simulink model "ctrl_ez0"  (R2024b)
settings: Solver=FixedStepDiscrete  StartTime=0.0  StopTime=10.0  RelTol=1e-3  EnableMultiTasking=on
InitFcn:
  | fidelity_pfc_vals;
values from neighbouring files (symbols this model uses):
  cos_th = cos(2*pi*50*t)    [fidelity_pfc_vals.m]
  sin_th = sin(2*pi*50*t)    [fidelity_pfc_vals.m]
  tsw = 1/(fsw*1e3)    (= 1.53846153846e-05)    [fidelity_pfc_vals.m]
undefined symbols (not defined in the file or in its folder): DiscIntNeverNeededParam
libraries: simulink x4, mcbcontrolslib x1, dspswit3 x1, slpidlib x1, simulink_extras x1
settings Model: DataDictionary=dic_pfc3ph.sldd  Creator=Angel  LastModifiedBy=Angel
settings DataIOCC: SaveOutput=off  SaveTime=off
settings OptimizationCC: DefaultParameterBehavior=Inlined  UseDivisionForNetSlopeComputation=on  GainParamInheritBuiltInType=on  UseFloatMulNetSlope=on  DefaultUnderspecifiedDataType=single  InlineInvariantSignals=on  ReuseModelBlockBuffer=off  PassReuseOutputArgsAs=Individual arguments  ZeroExternalMemoryAtStartup=off  ZeroInternalMemoryAtStartup=off  NoFixptDivByZeroProtection=on  EfficientFloat2IntCast=on  LifeSpan=1  BufferReusableBoundary=off  OptimizationLevel=level1  OptimizationPriority=Speed  EfficientTunableParamExpr=on
settings DebuggingCC: MergeDetectMultiDrivingBlocksExec=none  ParameterTunabilityLossMsg=error
settings HardwareCC: ProdBitPerPointer=32  ProdBitPerSizeT=32  ProdBitPerPtrDiffT=32  ProdLargestAtomicInteger=Long  ProdLargestAtomicFloat=Double  ProdWordSize=32  ProdLongLongMode=on  ProdHWDeviceType=ARM Compatible->ARM Cortex-M
settings ModelReferenceCC: ModelReferenceNumInstancesAllowed=Single  PropagateSignalLabelsOutOfModel=off
settings SFSimCC: MATLABDynamicMemAlloc=off
settings RTWCC: Description=Embedded Coder  SystemTargetFile=ert.tlc  EmbeddedCoderDictionary=dic_pfc3ph.sldd  GenCodeOnly=on  TemplateMakefile=ert_default_tmf  Toolchain=CMake  DataTypeReplacement=CDataTypesFixedWidth
settings CodeAppCC: ForceParamTrailComments=on  CommentStyle=Multi-line  IgnoreCustomStorageClasses=off  OperatorAnnotations=on  SimulinkDataObjDesc=on  SFDataObjDesc=on  CustomSymbolStrGlobalVar=rt$N$M  CustomSymbolStrType=$N$M  CustomSymbolStrFcn=$N$M$F  CustomSymbolStrMacro=$N$M  InsertBlockDesc=on
settings ERTTargetCC: IncludeMdlTerminateFcn=off  CombineSignalStateStructs=on  SupportAbsoluteTime=off  SupportComplex=off  SupportNonInlinedSFcns=on  RemoveResetFunc=off  ParenthesesLevel=Standards  RootIOFormat=Structure reference  ERTCustomFileTemplate=example_file_process.tlc  ERTFilePackagingFormat=CompactWithDataFile  MaxIdInt64=INT64_MAX  MinIdInt64=INT64_MIN  MaxIdUint64=UINT64_MAX  MaxIdInt32=INT32_MAX  MinIdInt32=INT32_MIN  MaxIdUint32=UINT32_MAX  MaxIdInt16=INT16_MAX  MinIdInt16=INT16_MIN  MaxIdUint16=UINT16_MAX  MaxIdInt8=INT8_MAX  MinIdInt8=INT8_MIN  MaxIdUint8=UINT8_MAX

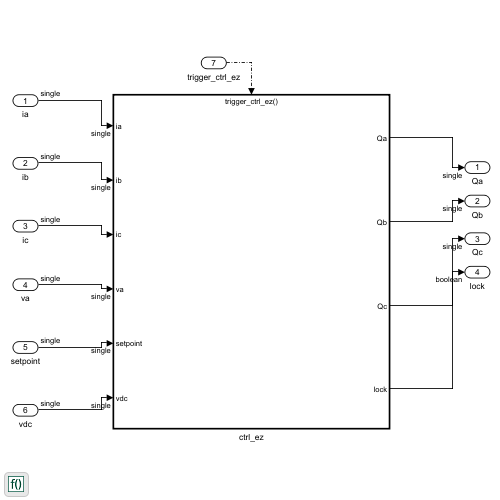
[thumbnail: Simulink's stored preview of the top-level diagram]
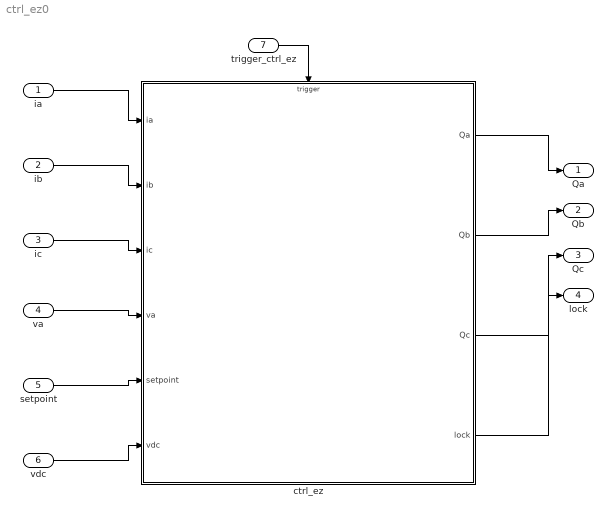
== system ctrl_ez0 ==
  ia : Inport  OutDataTypeStr=single  PortDimensions=1
  ib : Inport  Port=2  OutDataTypeStr=single  PortDimensions=1
  ic : Inport  Port=3  OutDataTypeStr=single  PortDimensions=1
  va : Inport  Port=4  OutDataTypeStr=single  PortDimensions=1
  setpoint : Inport  Port=5  OutDataTypeStr=single  PortDimensions=1
  vdc : Inport  Port=6  OutDataTypeStr=single  PortDimensions=1
  trigger_ctrl_ez : Inport  Port=7  PortDimensions=1  OutputFunctionCall=on
  ctrl_ez : Subsystem
  Qa : Outport  OutDataTypeStr=single  PortDimensions=1
  Qb : Outport  Port=2  OutDataTypeStr=single  PortDimensions=1
  Qc : Outport  Port=3  OutDataTypeStr=single  PortDimensions=1
  lock : Outport  Port=4  OutDataTypeStr=boolean  PortDimensions=1
  wires:
  ia/1 -> ctrl_ez/1(ia)
  ib/1 -> ctrl_ez/2(ib)
  ic/1 -> ctrl_ez/3(ic)
  va/1 -> ctrl_ez/4(va)
  setpoint/1 -> ctrl_ez/5(setpoint)
  vdc/1 -> ctrl_ez/6(vdc)
  ctrl_ez/1(Qa) -> Qa/1
  ctrl_ez/2(Qb) -> Qb/1
  ctrl_ez/3(Qc) -> Qc/1
  ctrl_ez/4(lock) -> lock/1
  trigger_ctrl_ez/1 -> ctrl_ez/Trigger

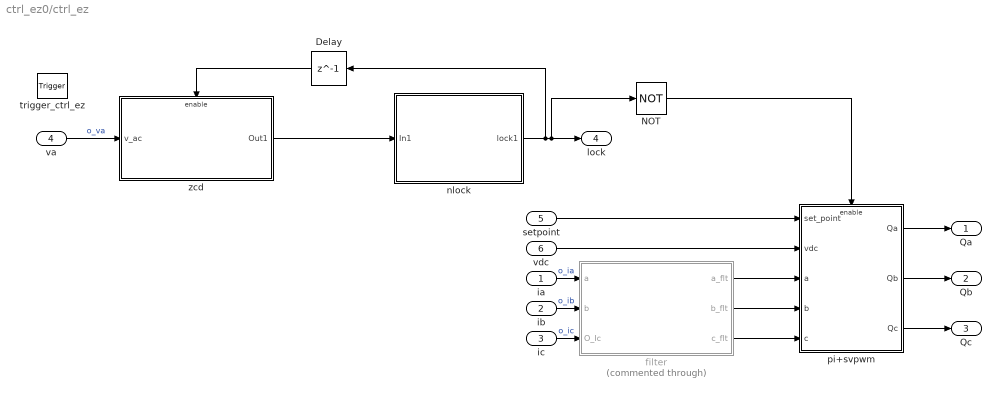
== system ctrl_ez0/ctrl_ez ==
  ia : Inport  OutDataTypeStr=single
  ib : Inport  Port=2  OutDataTypeStr=single
  ic : Inport  Port=3
  va : Inport  Port=4  OutDataTypeStr=single
  setpoint : Inport  Port=5  OutDataTypeStr=single
  vdc : Inport  Port=6  OutDataTypeStr=single
  trigger_ctrl_ez : TriggerPort  TriggerType=function-call  VariantControl=(inherit)  PortDimensions=1
  Delay : Delay  DelayLength=1
  NOT : Logic  Operator=NOT  IconShape=distinctive  AllPortsSameDT=off  OutDataTypeStr=boolean
  filter : Subsystem  Commented=through
  nlock : Subsystem
  pi+svpwm : Subsystem
  zcd : Subsystem  SystemSampleTime=tsw
  Qa : Outport
  Qb : Outport  Port=2
  Qc : Outport  Port=3
  lock : Outport  Port=4
  wires:
  pi+svpwm/3(Qc) -> Qc/1
  pi+svpwm/2(Qb) -> Qb/1
  pi+svpwm/1(Qa) -> Qa/1
  filter/2(b_flt) -> pi+svpwm/4(b)
  vdc/1 -> pi+svpwm/2(vdc)
  setpoint/1 -> pi+svpwm/1(set_point)
  filter/3(c_flt) -> pi+svpwm/5(c)
  nlock/1(lock1) -> Delay/1, NOT/1, lock/1
  zcd/1(Out1) -> nlock/1(In1)
  va/1 -> zcd/1(v_ac)  "o_va"
  filter/1(a_flt) -> pi+svpwm/3(a)
  Delay/1 -> zcd/Enable
  ia/1 -> filter/1(a)  "o_ia"
  ic/1 -> filter/3(O_Ic)  "o_ic"
  NOT/1 -> pi+svpwm/Enable
  ib/1 -> filter/2(b)  "o_ib"

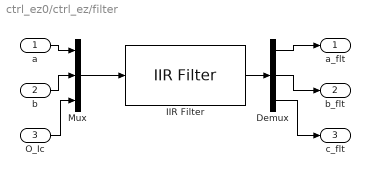
== system ctrl_ez0/ctrl_ez/filter ==
  a : Inport
  b : Inport  Port=2
  O_Ic : Inport  Port=3
  Demux : Demux  Outputs=3
  IIR Filter : mcbcontrolslib/IIR Filter  VariantControl=Low Pass Filter  VariantSelect=Low-pass  FilterConstantInputType=Specify via dialog  Filter_constant=.2  advancedSettings=on  Ts=tsw  cutOff_freq=2586.2678
  Mux : Mux  Inputs=3
  a_flt : Outport
  b_flt : Outport  Port=2
  c_flt : Outport  Port=3
  wires:
  Demux/3 -> c_flt/1
  O_Ic/1 -> Mux/3
  IIR Filter/1 -> Demux/1
  Demux/1 -> a_flt/1
  Mux/1 -> IIR Filter/1
  b/1 -> Mux/2
  Demux/2 -> b_flt/1
  a/1 -> Mux/1

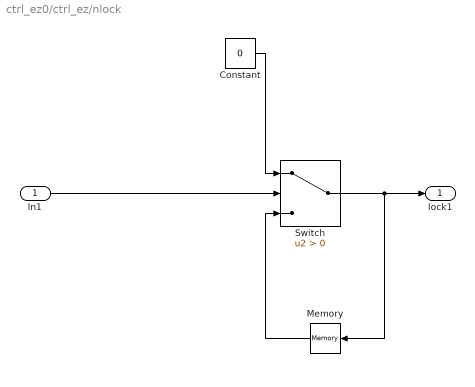
== system ctrl_ez0/ctrl_ez/nlock ==
  In1 : Inport
  Constant : Constant  Value=0  OutDataTypeStr=boolean  SampleTime=-1
  Memory : Memory  InitialCondition=1  InheritSampleTime=on
  Switch : Switch  Criteria=u2 > Threshold  SaturateOnIntegerOverflow=off  InputSameDT=off
  lock1 : Outport
  wires:
  In1/1 -> Switch/2
  Memory/1 -> Switch/3
  Constant/1 -> Switch/1
  Switch/1 -> Memory/1, lock1/1

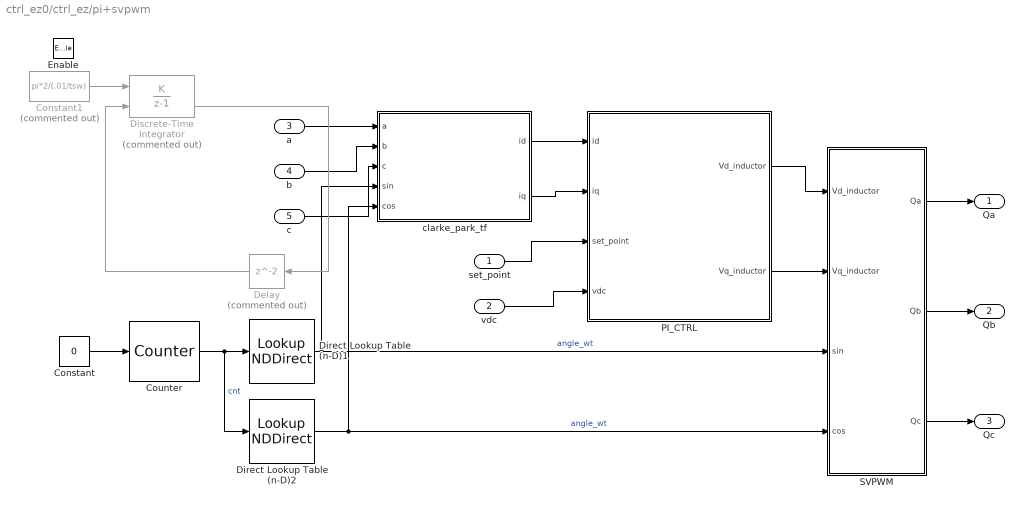
== system ctrl_ez0/ctrl_ez/pi+svpwm ==
  set_point : Inport
  vdc : Inport  Port=2
  a : Inport  Port=3
  b : Inport  Port=4
  c : Inport  Port=5
  Enable : EnablePort
  Constant : Constant  Value=0  SampleTime=-1
  Constant1 : Constant  Commented=on  Value=pi*2/(.01/tsw)  SampleTime=-1
  Counter : dspswit3/Counter  Direction=Up  CountEvent=Free running  CounterSize=User defined  MaxCount=(.01/tsw)+1  InitialCount=0  Output=Count  HitValue=32  ResetInput=on  SamplesPerFrame=1  Ts=-1  CntDtype=uint32  HitDtype=Logical
  Delay : Delay  Commented=on
  Direct Lookup Table (n-D)1 : LookupNDDirect  NumberOfTableDimensions=1  Table=single(sin_th);  RemoveProtectionInput=on  TableDataTypeStr=single
  Direct Lookup Table (n-D)2 : LookupNDDirect  NumberOfTableDimensions=1  Table=single(cos_th);  RemoveProtectionInput=on  TableDataTypeStr=single
  Discrete-Time Integrator : DiscreteIntegrator  Commented=on  IntegratorMethod=Accumulation: Forward Euler  gainval=1  ExternalReset=level  SampleTime=-1  SaturateOnIntegerOverflow=on  LimitOutput=on  UpperSaturationLimit=pi*2  ShowSaturationPort=on  ICPrevOutput=DiscIntNeverNeededParam  ICPrevScaledInput=DiscIntNeverNeededParam
  PI_CTRL : Subsystem  SystemSampleTime=tsw
  SVPWM : Subsystem  SystemSampleTime=tsw
  clarke_park_tf : Subsystem
  Qa : Outport
  Qb : Outport  Port=2
  Qc : Outport  Port=3
  wires:
  SVPWM/3(Qc) -> Qc/1
  SVPWM/2(Qb) -> Qb/1
  SVPWM/1(Qa) -> Qa/1
  PI_CTRL/2(Vq_inductor) -> SVPWM/2(Vq_inductor)
  vdc/1 -> PI_CTRL/4(vdc)
  set_point/1 -> PI_CTRL/3(set_point)
  clarke_park_tf/1(id) -> PI_CTRL/1(id)
  Direct Lookup Table (n-D)2/1 -> clarke_park_tf/5(cos), SVPWM/4(cos)  "angle_wt"
  Direct Lookup Table (n-D)1/1 -> clarke_park_tf/4(sin), SVPWM/3(sin)  "angle_wt"
  b/1 -> clarke_park_tf/2(b)
  Counter/1 -> Direct Lookup Table (n-D)1/1, Direct Lookup Table (n-D)2/1  "cnt"
  a/1 -> clarke_park_tf/1(a)
  c/1 -> clarke_park_tf/3(c)
  Constant/1 -> Counter/1
  clarke_park_tf/2(iq) -> PI_CTRL/2(iq)
  Delay/1 -> Discrete-Time Integrator/2
  PI_CTRL/1(Vd_inductor) -> SVPWM/1(Vd_inductor)
  Constant1/1 -> Discrete-Time Integrator/1
  Discrete-Time Integrator/2 -> Delay/1

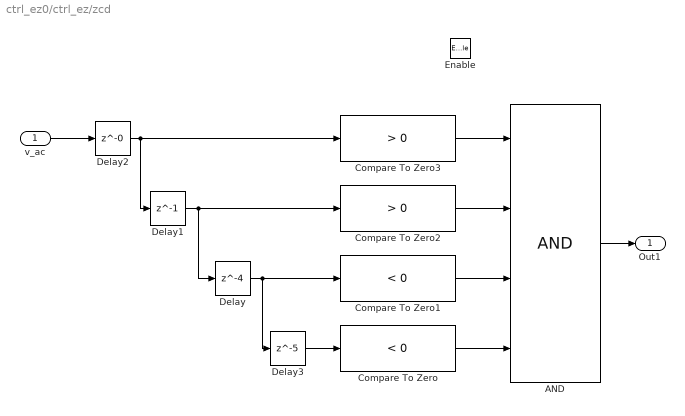
== system ctrl_ez0/ctrl_ez/zcd ==
  v_ac : Inport  OutDataTypeStr=single
  Enable : EnablePort
  AND : Logic  Inputs=4  AllPortsSameDT=off  OutDataTypeStr=boolean
  Compare To Zero : simulink/Logic and Bit Operations/Compare To Zero  relop=<  OutDataTypeStr=boolean
  Compare To Zero1 : simulink/Logic and Bit Operations/Compare To Zero  relop=<  OutDataTypeStr=boolean
  Compare To Zero2 : simulink/Logic and Bit Operations/Compare To Zero  relop=>  OutDataTypeStr=boolean
  Compare To Zero3 : simulink/Logic and Bit Operations/Compare To Zero  relop=>  OutDataTypeStr=boolean
  Delay : Delay  DelayLength=4
  Delay1 : Delay  DelayLength=1
  Delay2 : Delay  DelayLength=0
  Delay3 : Delay  DelayLength=5
  Out1 : Outport
  wires:
  AND/1 -> Out1/1
  Compare To Zero2/1 -> AND/2
  Compare To Zero/1 -> AND/4
  Compare To Zero1/1 -> AND/3
  Compare To Zero3/1 -> AND/1
  Delay1/1 -> Delay/1, Compare To Zero2/1
  Delay2/1 -> Delay1/1, Compare To Zero3/1
  Delay/1 -> Compare To Zero1/1, Delay3/1
  Delay3/1 -> Compare To Zero/1
  v_ac/1 -> Delay2/1

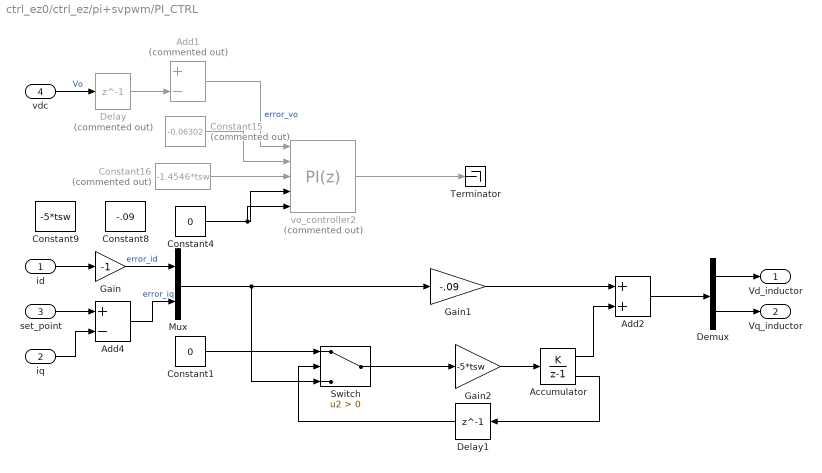
== system ctrl_ez0/ctrl_ez/pi+svpwm/PI_CTRL ==
  id : Inport
  iq : Inport  Port=2  OutDataTypeStr=single
  set_point : Inport  Port=3
  vdc : Inport  Port=4
  Accumulator : DiscreteIntegrator  IntegratorMethod=Accumulation: Forward Euler  SampleTime=-1  UpperSaturationLimit=50  LowerSaturationLimit=-50  ShowSaturationPort=on  ICPrevOutput=DiscIntNeverNeededParam  ICPrevScaledInput=DiscIntNeverNeededParam
  Add1 : Sum  Commented=on  Inputs=+-
  Add2 : Sum
  Add4 : Sum  Inputs=+-
  Constant1 : Constant  Value=0  OutDataTypeStr=single  SampleTime=-1
  Constant15 : Constant  Commented=on  Value=-0.06302  OutDataTypeStr=single  SampleTime=-1
  Constant16 : Constant  Commented=on  Value=-1.4546*tsw  OutDataTypeStr=single  SampleTime=-1
  Constant4 : Constant  Value=0  OutDataTypeStr=single  SampleTime=-1
  Constant8 : Constant  Value=-.09  OutDataTypeStr=single  SampleTime=-1
  Constant9 : Constant  Value=-5*tsw  OutDataTypeStr=single  SampleTime=-1
  Delay : Delay  Commented=on  DelayLength=1  InitialCondition=580
  Delay1 : Delay  DelayLength=1  InputProcessing=Columns as channels (frame based)
  Demux : Demux  Outputs=2
  Gain : Gain  Gain=-1  OutDataTypeStr=single
  Gain1 : Gain  Gain=-.09  OutDataTypeStr=single
  Gain2 : Gain  Gain=-5*tsw  OutDataTypeStr=single
  Mux : Mux  Inputs=2
  Switch : Switch  Criteria=u2 > Threshold  SaturateOnIntegerOverflow=off  InputSameDT=off
  Terminator : Terminator
  vo_controller2 : slpidlib/PID Controller  Commented=on  Controller=PI  Form=Parallel  TimeDomain=Discrete-time  UseExternalTs=on  SampleTime=-1  IntegratorMethod=Forward Euler  FilterMethod=Forward Euler  ControllerParametersSource=external  P=-0.053025  I=-1.4546  UseKiTs=on  D=0  UseExternalDerivativeSource=off  N=100  UseFilter=on  TunerSelectOption=Transfer Function Based (PID Tuner App)  InitialConditionSource=external  InitialConditionForIntegrator=0  InitialConditionForFilter=0  DifferentiatorICPrevScaledInput=0  ExternalReset=level  TrackingMode=off  Kt=1  LimitOutput=on  SatLimitsSource=internal  UpperSaturationLimit=300  LowerSaturationLimit=-300  LinearizeAsGain=on  AntiWindupMode=clamping  Kb=1  LimitIntegrator=off  UpperIntegratorSaturationLimit=inf  LowerIntegratorSaturationLimit=-inf  POutMin=[]  POutMax=[]  IOutMin=[]  IOutMax=[]  DOutMin=[]  DOutMax=[]  NOutMin=[]  NOutMax=[]  SumOutMin=[]  SumOutMax=[]  SaturationOutMin=[]  SaturationOutMax=[]  PParamMin=[]  PParamMax=[]  IParamMin=[]  IParamMax=[]  DParamMin=[]  DParamMax=[]  NParamMin=[]  NParamMax=[]  KbParamMin=[]  KbParamMax=[]  KtParamMin=[]  KtParamMax=[]  KbOutMin=[]  KbOutMax=[]  KtOutMin=[]  KtOutMax=[]  IntegratorOutMin=[]  IntegratorOutMax=[]  FilterOutMin=[]  FilterOutMax=[]  SumI1OutMin=[]  SumI1OutMax=[]  SumI2OutMin=[]  SumI2OutMax=[]  SumI3OutMin=[]  SumI3OutMax=[]  SumI4OutMin=[]  SumI4OutMax=[]  SumDOutMin=[]  SumDOutMax=[]  DifferentiatorOutMin=[]  DifferentiatorOutMax=[]  FilterDiffOutCoefMin=[]  FilterDiffOutCoefMax=[]  ReciprocalOutMin=[]  ReciprocalOutMax=[]  SumDenOutMin=[]  SumDenOutMax=[]  SumNumOutMin=[]  SumNumOutMax=[]  DivideOutMin=[]  DivideOutMax=[]  UdiffTsProdOutMin=[]  UdiffTsProdOutMax=[]  NTsProdOutMin=[]  NTsProdOutMax=[]  UintegralTsProdOutMin=[]  UintegralTsProdOutMax=[]  UngainTsProdOutMin=[]  UngainTsProdOutMax=[]  ClampingZeroOutDataTypeStr=Inherit: Inherit via back propagation  ClampingZeroOutMin=[]  ClampingZeroOutMax=[]  FilterDenConstantOutDataTypeStr=Inherit: Inherit via back propagation  FilterDenConstantOutMin=[]  FilterDenConstantOutMax=[]  PCopyOutDataTypeStr=Inherit: Inherit via back propagation  PCopyOutMin=[]  PCopyOutMax=[]  NCopyOutDataTypeStr=Inherit: Inherit via back propagation  NCopyOutMin=[]  NCopyOutMax=[]  IntegratorContinuousStateAttributes=''  IntegratorStateMustResolveToSignalObject=off  IntegratorRTWStateStorageClass=Auto  FilterContinuousStateAttributes=''  FilterStateMustResolveToSignalObject=off  FilterRTWStateStorageClass=Auto  ParallelPVariant=ExternalParameters  IdealPVariant=Disabled  IVariant=ExternalParameters  DVariant=Disabled  IntegratorVariant=Discrete  SatVariant=Enabled  AWVariant=DiscClampingParallel  PCopyVariant=Disabled  TRVariant=Disabled  FdbkBlocksVariant=Forward  IdealPFdbkVariant=Disabled  SatFdbkVariant=Disabled  DerivativeFilterVariant=Disabled  NVariant=Disabled  NCopyVariant=Disabled_SignalSpec  FilterICVariant=Disabled  IntegratorICVariant=ExternalICs  ExternalResetVariant=ExternalReset  TRSumVariant=Passthrough  SumFdbkVariant=Disabled  SumVariant=Sum_PI  TsampFilterVariant=InternalTs  TsampNgainVariant=Passthrough  TsampIntegralVariant=Passthrough  ExternalSaturationOutDataTypeStr=Inherit: Same as second input  DerivativeSourceVariant=Disabled  PreIntVariant=InternalPreInt
  Vd_inductor : Outport
  Vq_inductor : Outport  Port=2
  wires:
  Demux/2 -> Vq_inductor/1
  Accumulator/2 -> Delay1/1
  Accumulator/1 -> Add2/2
  Gain2/1 -> Accumulator/1
  Delay1/1 -> Switch/2
  Switch/1 -> Gain2/1
  vo_controller2/1 -> Terminator/1
  Constant1/1 -> Switch/1
  Mux/1 -> Switch/3, Gain1/1
  Constant4/1 -> vo_controller2/5, vo_controller2/4
  Constant16/1 -> vo_controller2/3
  Constant15/1 -> vo_controller2/2
  Gain/1 -> Mux/1  "error_id"
  Add2/1 -> Demux/1
  Add4/1 -> Mux/2  "error_iq"
  Add1/1 -> vo_controller2/1  "error_vo"
  Demux/1 -> Vd_inductor/1
  iq/1 -> Add4/2
  set_point/1 -> Add4/1
  Gain1/1 -> Add2/1
  id/1 -> Gain/1
  vdc/1 -> Delay/1  "Vo"
  Delay/1 -> Add1/2

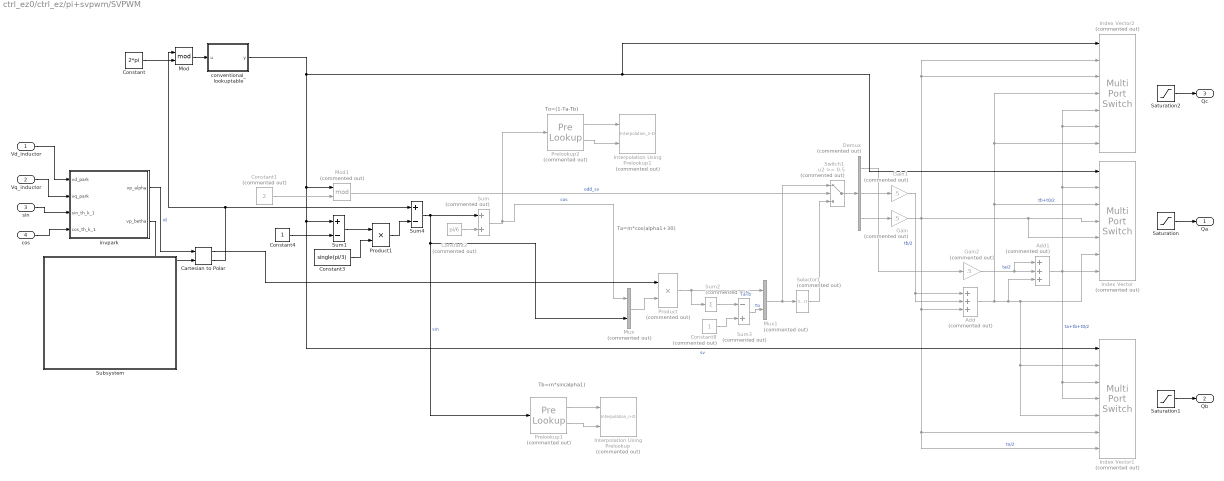
== system ctrl_ez0/ctrl_ez/pi+svpwm/SVPWM ==
  note: To=(1-Ta-Tb)
  note: Ta=m*cos(alpha1+30)
  note: Tb=m*sin(alpha1)
  Vd_inductor : Inport
  Vq_inductor : Inport  Port=2
  sin : Inport  Port=3
  cos : Inport  Port=4
  Add : Sum  Commented=on  Inputs=+++
  Add1 : Sum  Commented=on  Inputs=+++
  Cartesian to Polar : simulink_extras/Transformations/Cartesian to Polar
  Constant : Constant  Value=2*pi  OutDataTypeStr=single  SampleTime=-1
  Constant1 : Constant  Commented=on  Value=2  OutDataTypeStr=single  SampleTime=-1
  Constant2 : Constant  Commented=on  Value=pi/6  OutDataTypeStr=single  SampleTime=-1
  Constant3 : Constant  Value=single(pi/3)  VectorParams1D=off  OutDataTypeStr=single  SampleTime=-1
  Constant4 : Constant  OutDataTypeStr=single  SampleTime=-1
  Constant8 : Constant  Commented=on  OutDataTypeStr=single  SampleTime=-1
  Demux : Demux  Commented=on  Outputs=3
  Gain : Gain  Commented=on  Gain=.5  OutDataTypeStr=single
  Gain1 : Gain  Commented=on  Gain=.5  OutDataTypeStr=single
  Gain2 : Gain  Commented=on  Gain=.5  OutDataTypeStr=single
  Index Vector : MultiPortSwitch  Commented=on  Inputs=6  DiagnosticForDefault=None  SaturateOnIntegerOverflow=off  InputSameDT=off
  Index Vector1 : MultiPortSwitch  Commented=on  Inputs=6  DiagnosticForDefault=None  SaturateOnIntegerOverflow=off  InputSameDT=off
  Index Vector2 : MultiPortSwitch  Commented=on  Inputs=6  DiagnosticForDefault=None  SaturateOnIntegerOverflow=off  InputSameDT=off
  Interpolation Using Prelookup : Interpolation_n-D  Commented=on  NumberOfTableDimensions=1  Table=single(sin(0:2*pi/1024:2*pi))  InterpMethod=Flat  RemoveProtectionIndex=on  ValidIndexMayReachLast=on  InternalRulePriority=Speed
      settings: InputPortMap=u0,u1
  Interpolation Using Prelookup1 : Interpolation_n-D  Commented=on  NumberOfTableDimensions=1  Table=single(cos(0:2*pi/1024:2*pi))  InterpMethod=Flat  RemoveProtectionIndex=on  ValidIndexMayReachLast=on  InternalRulePriority=Speed
      settings: InputPortMap=u0,u1
  Mod : Math  Operator=mod
  Mod1 : Math  Commented=on  Operator=mod
  Mux : Mux  Commented=on  Inputs=2
  Mux1 : Mux  Commented=on  Inputs=2
  Prelookup1 : PreLookup  Commented=on  BreakpointsData=single((0:2*pi/1024:2*pi))  IndexSearchMethod=Evenly spaced points  BeginIndexSearchUsingPreviousIndexResult=on  UseLastBreakpoint=on
  Prelookup2 : PreLookup  Commented=on  BreakpointsData=single((0:2*pi/1024:2*pi))  IndexSearchMethod=Evenly spaced points  BeginIndexSearchUsingPreviousIndexResult=on  UseLastBreakpoint=on
  Product : Product  Commented=on  SaturateOnIntegerOverflow=on  OutDataTypeStr=Inherit: Same as first input
  Product1 : Product  OutDataTypeStr=single
  Saturation : Saturate  UpperLimit=.98  LowerLimit=.03
  Saturation1 : Saturate  UpperLimit=.98  LowerLimit=.03
  Saturation2 : Saturate  UpperLimit=.98  LowerLimit=.03
  Selector1 : Selector  Commented=on  InputPortWidth=3  IndexOptions=Index vector (dialog)  Indices=[2 1 3]  OutputSizes=1
  Subsystem : Subsystem
  Sum : Sum  Commented=on  SaturateOnIntegerOverflow=on
  Sum1 : Sum  Inputs=+-  SaturateOnIntegerOverflow=on
  Sum2 : Sum  Commented=on  Inputs=1  SaturateOnIntegerOverflow=on
  Sum3 : Sum  Commented=on  Inputs=-+  SaturateOnIntegerOverflow=on
  Sum4 : Sum  Inputs=+-  SaturateOnIntegerOverflow=on
  Switch1 : Switch  Commented=on  Threshold=0.5  InputSameDT=off
  conventional_lookuptable : MATLAB Function  TreatAsAtomicUnit=on
  invpark : MATLAB Function  TreatAsAtomicUnit=on  VariantControl=false()
  Qa : Outport
  Qb : Outport  Port=2
  Qc : Outport  Port=3
  wires:
  Vq_inductor/1 -> invpark/2(vq_park)
  Prelookup2/1 -> Interpolation Using Prelookup1/1
  Prelookup2/2 -> Interpolation Using Prelookup1/2
  Prelookup1/2 -> Interpolation Using Prelookup/2
  Prelookup1/1 -> Interpolation Using Prelookup/1
  Mod/1 -> conventional_lookuptable/1(u)
  invpark/1(vp_alpha) -> Cartesian to Polar/1  "id"
  invpark/2(vp_betha) -> Cartesian to Polar/2
  Vd_inductor/1 -> invpark/1(vd_park)
  cos/1 -> invpark/4(cos_th_k_1)
  sin/1 -> invpark/3(sin_th_k_1)
  Saturation1/1 -> Qb/1
  Saturation/1 -> Qa/1
  Saturation2/1 -> Qc/1
  Add1/1 -> Index Vector/7, Index Vector/2, Index Vector2/6, Index Vector2/5, Index Vector1/3, Index Vector1/4  "ta+tb+t0/2"
  Add/1 -> Index Vector/3, Index Vector2/7, Index Vector2/4, Add1/3, Index Vector/6, Index Vector1/2, Index Vector1/5  "tb+t0/2"
  Gain2/1 -> Add1/2, Add1/1  "ta/2"
  Gain/1 -> Index Vector2/2, Index Vector2/3, Index Vector/4, Index Vector/5, Add/3, Index Vector1/6, Index Vector1/7  "to/2"
  Demux/3 -> Gain/1
  Switch1/1 -> Demux/1
  Selector1/1 -> Switch1/3
  Mux1/1 -> Selector1/1, Switch1/1
  Sum3/1 -> Mux1/2  "To"
  Constant8/1 -> Sum3/2
  Sum2/1 -> Sum3/1
  Product/1 -> Sum2/1, Mux1/1  "TaTb"
  Mux/1 -> Product/2
  Sum/1 -> Mux/1, Prelookup2/1  "cos"
  Sum4/1 -> Sum/1, Prelookup1/1, Mux/2  "sin"
  Demux/1 -> Gain2/1
  Constant2/1 -> Sum/2
  Product1/1 -> Sum4/2
  Constant3/1 -> Product1/2
  Sum1/1 -> Product1/1
  Mod1/1 -> Switch1/2  "odd_sv"
  Constant4/1 -> Sum1/2
  conventional_lookuptable/1(y) -> Index Vector/1, Index Vector2/1, Mod1/1, Sum1/1, Index Vector1/1  "sv"
  Constant1/1 -> Mod1/2
  Cartesian to Polar/1 -> Product/1
  Gain1/1 -> Add/2, Add/1  "tb/2"
  Constant/1 -> Mod/2
  Demux/2 -> Gain1/1
  Cartesian to Polar/2 -> Sum4/1, Mod/1

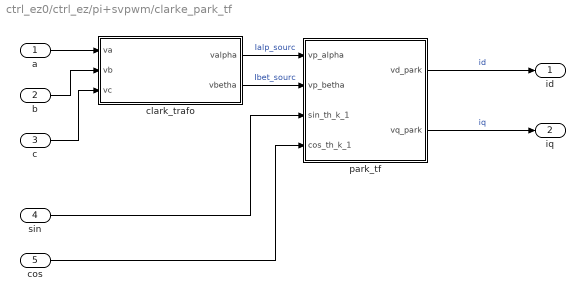
== system ctrl_ez0/ctrl_ez/pi+svpwm/clarke_park_tf ==
  a : Inport
  b : Inport  Port=2
  c : Inport  Port=3
  sin : Inport  Port=4
  cos : Inport  Port=5
  clark_trafo : MATLAB Function  TreatAsAtomicUnit=on
  park_tf : MATLAB Function  TreatAsAtomicUnit=on  VariantControl=false()
  id : Outport
  iq : Outport  Port=2
  wires:
  cos/1 -> park_tf/4(cos_th_k_1)
  sin/1 -> park_tf/3(sin_th_k_1)
  clark_trafo/2(vbetha) -> park_tf/2(vp_betha)  "Ibet_sourc"
  clark_trafo/1(valpha) -> park_tf/1(vp_alpha)  "Ialp_sourc"
  park_tf/2(vq_park) -> iq/1  "iq"
  park_tf/1(vd_park) -> id/1  "id"
  c/1 -> clark_trafo/3(vc)
  b/1 -> clark_trafo/2(vb)
  a/1 -> clark_trafo/1(va)

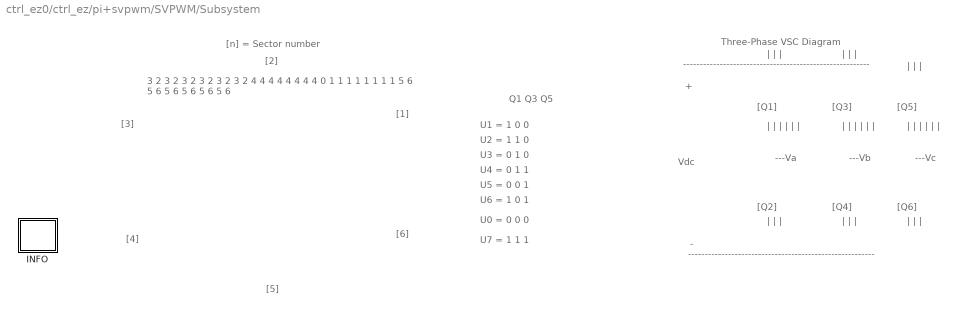
== system ctrl_ez0/ctrl_ez/pi+svpwm/SVPWM/Subsystem ==
  note: |
      | |
      | |
      | |
      | |
      | |
  note: +
  note: ---Vb
  note: --------------------------------------------------------
  note: |
      | |
      | |
  note: [4]
  note: |
      | |
      | |
  note: U0 = 0 0 0
  note: ---Vc
  note: [Q2]
  note: U2 = 1 1 0
  note: [Q1]
  note: [n] = Sector number
  note: U1 = 1 0 0
  note: |
      | |
      | |
      | |
      | |
      | |
  note: |
      | |
      | |
  note: [6]
  note: [1]
  note: [3]
  note: U6 = 1 0 1
  note: U4 = 0 1 1
  note: [2]
  note: |
      | |
      | |
  note: |
      | |
      | |
  note: 3                       2
      |       3                   2
      |         3               2
      |           3           2
      |             3       2
      |               3   2
      | 4 4 4 4 4 4 4 4 0 1 1 1 1 1 1 1 1
      |               5   6
      |             5       6
      |           5           6
      |         5               6
      |       5                   6
      |     5                       6
  note: [5]
  note: Vdc
  note: U5 = 0 0 1
  note: ---Va
  note: U3 = 0 1 0
  note: [Q3]
  note: [Q4]
  note: [Q5]
  note: [Q6]
  note: |
      | |
      | |
      | |
      | |
      | |
  note: |
      | |
      | |
  note: -
  note: Q1 Q3 Q5
  note: --------------------------------------------------------
  note: U7 = 1 1 1
  note: Three-Phase VSC Diagram
  INFO : Subsystem
      mask Display: disp('?')

== system ctrl_ez0/ctrl_ez/pi+svpwm/SVPWM/Subsystem/INFO ==
  note: Two symmetrical switching patterns have been implemented:
  note: 3                       2
      |       3                   2
      |         3               2
      |           3           2
      |             3       2
      |               3   2
      | 4 4 4 4 4 4 4 4 0 1 1 1 1 1 1 1 1
      |               5   6
      |             5       6
      |           5           6
      |         5               6
      |       5                   6
      |     5                       6
  note: [1]
  note: [3]
  note: [4]
  note: [5]
  note: [6]
  note: U1 = 1 0 0
  note: U2 = 1 1 0
  note: U3 = 0 1 0
  note: U0 = 0 0 0
  note: U6 = 1 0 1
  note: U5 = 0 0 1
  note: U4 = 0 1 1
  note: Basic Space Vectors and Switching States
  note: [2]
  note: [n] = Sector number
  note: Vdc
  note: [Q1]
  note: [Q2]
  note: |
      | |
      | |
      | |
      | |
      | |
  note: |
      | |
      | |
  note: ---Va
  note: |
      | |
      | |
  note: [Q3]
  note: [Q4]
  note: |
      | |
      | |
      | |
      | |
      | |
  note: |
      | |
      | |
  note: ---Vb
  note: |
      | |
      | |
  note: [Q5]
  note: [Q6]
  note: |
      | |
      | |
      | |
      | |
      | |
  note: |
      | |
      | |
  note: ---Vc
  note: |
      | |
      | |
  note: --------------------------------------------------------
  note: +
  note: -
  note: Three-Phase VSC Diagram
  note: --------------------------------------------------------
  note: Q1 Q3 Q5
  note: U7 = 1 1 1
  note: The objective of the SV PWM technique is to approximate the reference voltage vector (U*) instantaneously
      | by combination of the switching states corresponding to the basic space vectors.
  note: Reference: Application Report SPRA524
      | Space-Vector PWM with TMS320C24x Using H/W & S/W Determined Switching Patterns
      | Zhenyu Yu, Texas Instruments
  note: --------------------------------------------------------------------------------------------------------------------------------------------------------------------
  note: Pattern #1:
      | With this pattern, identified as "Software-Determined" by Texas Instruments, each PWM channel switches twice per every PWM period.
  note: Pattern #2:
      | With this pattern, identified as "Hardware-Determined" by Texas Instruments, there is always one PWM channel staying constant for the entire PWM period.
      |  So the number of switching times for this pattern is less than pattern #1. As a result, switching losses will be reduced with Pattern #2.

== matlab function ctrl_ez0/ctrl_ez/pi+svpwm/SVPWM/invpark ==
  data: vp_alpha output; vd_park input; vq_park input; sin_th_k_1 input; cos_th_k_1 input; vp_betha output
function [vp_alpha,vp_betha]  = invpark(vd_park,vq_park,sin_th_k_1,cos_th_k_1)

%vq_park=(sin_th_k_1*vp_betha+cos_th_k_1*vp_alpha);%(-sin_th_k_1*vp_alpha+cos_th_k_1*vp_betha);
%vd_park=(sin_th_k_1*vp_alpha-cos_th_k_1*vp_betha);
%vp_betha= (cos_th_k_1*vp_alpha - vq_park) /  sin_th_k_1
%vd_park+cos_th_k_1*vp_betha = sin_th_k_1*vp_alpha
%vd_park + cos_th_k_1 * (cos_th_k_1*vp_alpha - vq_park) /  sin_th_k_1 = sin_th_k_1*vp_alpha
%vd_park * sin_th_k_1 + cos_th_k_1 * (cos_th_k_1*vp_alpha - vq_park) = sin_th_k_1*sin_th_k_1*vp_alpha
%vd_park * sin_th_k_1 +cos_th_k_1*cos_th_k_1*vp_alpha - cos_th_k_1*vq_park= sin_th_k_1*sin_th_k_1*vp_alpha
%vd_park * sin_th_k_1- cos_th_k_1*vq_park= sin_th_k_1*sin_th_k_1*vp_alpha-cos_th_k_1*cos_th_k_1*vp_alpha
%vd_park * sin_th_k_1- cos_th_k_1*vq_park= (sin_th_k_1*sin_th_k_1-cos_th_k_1*cos_th_k_1)*vp_alpha
% vp_alpha = ((vd_park * sin_th_k_1)-( cos_th_k_1*vq_park)) /
% ((sin_th_k_1*sin_th_k_1)-(cos_th_k_1*cos_th_k_1))
vp_alpha = ((vd_park * sin_th_k_1)-( cos_th_k_1*vq_park)) / ((sin_th_k_1*sin_th_k_1)-(cos_th_k_1*cos_th_k_1));
vp_betha = (cos_th_k_1*vp_alpha - vq_park) /  sin_th_k_1;
end

== matlab function ctrl_ez0/ctrl_ez/pi+svpwm/SVPWM/conventional_lookuptable ==
  data: u input single; y output single
function y = fcn(u)

switch u
    case u>=single(0) && u<single(pi/3)
        y=single(1);
    case u>=single(pi/3) && u<single(2*pi/3)
        y=single(2);
    case u>=single(2*pi/3) && u<single(pi)
        y=single(3);
    case u>=single(pi) && u<single(4*pi/3)
        y=single(4);
    case u>=single(4*pi/3) && u<single(5*pi/3)
        y=single(5);
    case u>=single(5*pi/3) && u<single(2*pi)
        y=single(6);        
    otherwise
        y=single(1);


end

== matlab function ctrl_ez0/ctrl_ez/pi+svpwm/clarke_park_tf/clark_trafo ==
  settings: updateMethod=DISCRETE
  data: va input; valpha output; vb input; vc input; vbetha output
function [valpha, vbetha] = clarktrans(va,vb,vc)


valpha=((2/3)*(va-(.5*vb)-(.5*vc)));
vbetha=( ((2/3)*(sqrt(3)*.5))*(vb-vc) );

end

== matlab function ctrl_ez0/ctrl_ez/pi+svpwm/clarke_park_tf/park_tf ==
  data: vd_park output; vp_alpha input; vq_park output; vp_betha input; sin_th_k_1 input; cos_th_k_1 input
 function [vd_park,vq_park] = park(vp_alpha,vp_betha,sin_th_k_1,cos_th_k_1)

vq_park=(sin_th_k_1*vp_betha+cos_th_k_1*vp_alpha);%(-sin_th_k_1*vp_alpha+cos_th_k_1*vp_betha);
vd_park=(sin_th_k_1*vp_alpha-cos_th_k_1*vp_betha);


end
